simulink library "PV_lib"  (R2026a)
settings: Solver=VariableStepAuto
libraries: fl_lib x2, nesl_utility x2

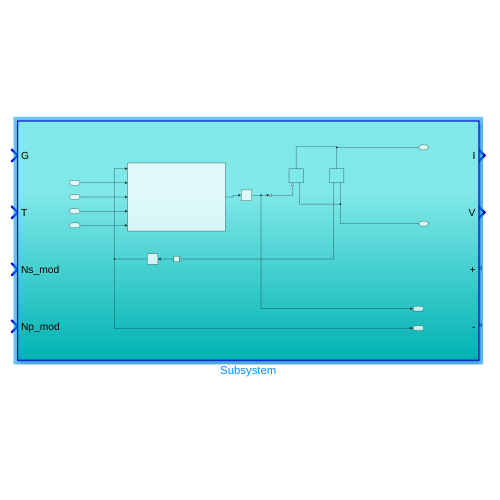
[thumbnail: Simulink's stored preview of the top-level diagram]
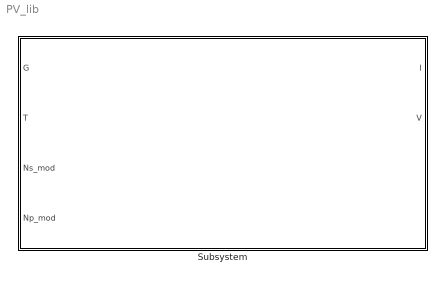
== system PV_lib ==
  Subsystem : Subsystem

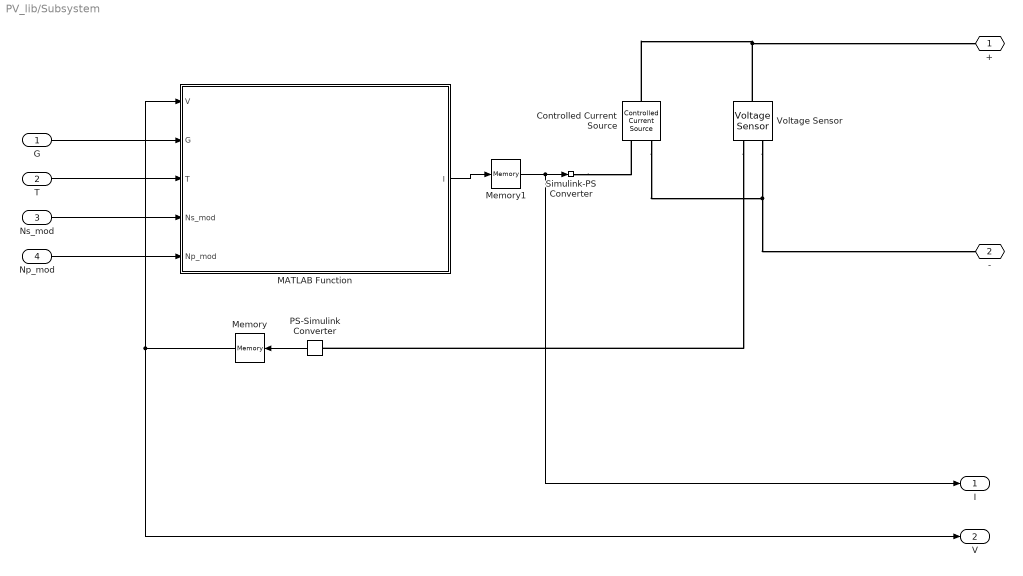
== system PV_lib/Subsystem ==
  G : Inport
  T : Inport  Port=2
  Ns_mod : Inport  Port=3
  Np_mod : Inport  Port=4
  Controlled Current Source : fl_lib/Electrical/Electrical Sources/Controlled Current Source
  MATLAB Function : MATLAB Function  TreatAsAtomicUnit=on
  Memory : Memory
  Memory1 : Memory
  PS-Simulink Converter : nesl_utility/PS-Simulink Converter  PhysicalDomain=network_engine_domain  SubClassName=ps_output  LeftPortType=input  RightPortType=output  PseudoPeriodic=off  Frequencies=[]  VectorFormat=inherit  Unit=inherit  AffineConversion=off
  Simulink-PS Converter : nesl_utility/Simulink-PS Converter  PhysicalDomain=network_engine_domain  SubClassName=ps_input  LeftPortType=input  RightPortType=output  PseudoPeriodic=off  Frequencies=[]  NoiseDistribution=none  NoiseParameters=[]  Unit=1  AffineConversion=off  FilteringAndDerivatives=provide  SimscapeFilterOrder=1  InputFilterTimeConstant=0.001  UdotUserProvided=0
  Voltage Sensor : fl_lib/Electrical/Electrical Sensors/Voltage Sensor
  + : PMIOPort  Side=Right
  - : PMIOPort  Port=2  Side=Right
  I : Outport
  V : Outport  Port=2
  wires:
  PS-Simulink Converter/1 -> Memory/1
  Memory/1 -> V/1, MATLAB Function/1(V)
  MATLAB Function/1(I) -> Memory1/1
  Memory1/1 -> I/1, Simulink-PS Converter/1
  G/1 -> MATLAB Function/2(G)
  T/1 -> MATLAB Function/3(T)
  Ns_mod/1 -> MATLAB Function/4(Ns_mod)
  Np_mod/1 -> MATLAB Function/5(Np_mod)
  connections:
  Simulink-PS Converter/RConn1 -- Controlled Current Source/RConn1
  Voltage Sensor/RConn1 -- PS-Simulink Converter/LConn1
  Controlled Current Source/RConn2 -- Voltage Sensor/RConn2 -- -/RConn1
  Controlled Current Source/LConn1 -- Voltage Sensor/LConn1 -- +/RConn1

== matlab function PV_lib/Subsystem/MATLAB Function ==
  data: I output; V input; G input; T input; Ns_mod input; Np_mod input
function I = modelo_pv(V,G,T,Ns_mod,Np_mod)
    % ---- Parâmetros de catálogo de UM painel (monocristalino, ~50W) ----
    Isc_ref_1 = 3.14;
    Voc_ref_1 = 21.4;
    Kv_1 = -0.080;
    Ki_1 = 0.0024;
    Ns_1 = 36;
    k = 1.3806e-23;
    q = 1.6022e-19;
    a = 1.2;

    % ---- Escala pro arranjo (Ns_mod em série, Np_mod em paralelo) ----
    Isc_ref = Isc_ref_1 * Np_mod;
    Voc_ref = Voc_ref_1 * Ns_mod;
    Kv = Kv_1 * Ns_mod;
    Ki = Ki_1 * Np_mod;
    Ns = Ns_1 * Ns_mod;

    T_kelvin = T + 273.15;
    T_ref = 25 + 273.15;
    G_ref = 1000;
    V = max(min(V, 1.5*Voc_ref), -1);
    Iph = (Isc_ref + Ki * (T_kelvin - T_ref)) * (G / G_ref);
    Irs = Isc_ref / (exp((q * Voc_ref) / (Ns * k * a * T_ref)) - 1);
    I0 = Irs * (T_kelvin / T_ref)^3 * exp((q * 1.12 / (a * k)) * (1/T_ref - 1/T_kelvin));
    expoente = min((q * V) / (Ns * k * a * T_kelvin), 80);
    Id = I0 * (exp(expoente) - 1);
    I = Iph - Id;
    if I < 0
        I = 0;
    end
end
